simulink model "arm_nonlinear_sim_pi_d_cont_MATLAB_function"  (R2019b)
settings: Solver=ode4  StartTime=0.0  StopTime=3  FixedStep=0.001  RelTol=1e-3
values from neighbouring files (symbols this model uses):
  c = 0.695    [arm_para.m]
  dc = 2    [arm_nonlinear_pi_d_design_MATLAB_function.m]
  g = 9.81    [arm_para.m]
  J = 0.0712    [arm_para.m]
  kD = (d2*gamma_m1^2 - d1*gamma_m1*gamma_m2                    + d0*(gamma_m2^2 - gamma_m1*gamma_m3))/(gamma_m1*gamma_m2)    [arm_nonlinear_pi_d_design_MATLAB_function.m]
  kI = d0/gamma_m1    [arm_nonlinear_pi_d_design_MATLAB_function.m]
  kP = (d2*gamma_m1 - d0*gamma_m3)/(gamma_m1*gamma_m2)    [arm_nonlinear_pi_d_design_MATLAB_function.m]
  l = 0.204    [arm_para.m]
  M = 0.390    (= 0.39)    [arm_para.m]
  rc = rc_deg*(pi/180)    (= 2.09439510239)    [arm_nonlinear_pi_d_design_MATLAB_function.m]
settings Model: Creator=kawata  LastModifiedBy=kawata
settings DataIOCC: ReturnWorkspaceOutputs=off
settings DebuggingCC: ArithmeticOperatorsInVariantConditions=warning
settings SFSimCC: SimUseLocalCustomCode=off  CustomCodeUndefinedFunction=UseInterfaceOnly
settings RTWCC: RTWUseLocalCustomCode=off

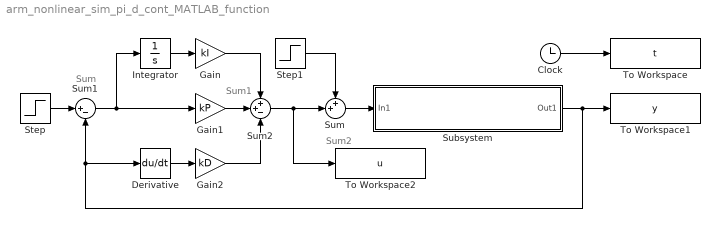
== system arm_nonlinear_sim_pi_d_cont_MATLAB_function ==
  note: Sum1
  note: Sum2
  note: Sum
  Clock : Clock
  Derivative : Derivative
  Gain : Gain  Gain=kI
  Gain1 : Gain  Gain=kP
  Gain2 : Gain  Gain=kD
  Integrator : Integrator
  Step : Step  Time=0  After=rc  SampleTime=0
  Step1 : Step  Time=1.5  After=dc  SampleTime=0
  Subsystem : Subsystem
  Sum : Sum  Inputs=++|
  Sum1 : Sum  Inputs=|+-
  Sum2 : Sum  Inputs=++-
  To Workspace : ToWorkspace  VariableName=t  SampleTime=-1
  To Workspace1 : ToWorkspace  VariableName=y  SampleTime=-1
  To Workspace2 : ToWorkspace  VariableName=u  SampleTime=-1
  wires:
  Subsystem/1(Out1) -> To Workspace1/1, Derivative/1, Sum1/2
  Clock/1 -> To Workspace/1
  Step/1 -> Sum1/1
  Sum/1 -> Subsystem/1(In1)
  Step1/1 -> Sum/1
  Sum2/1 -> To Workspace2/1, Sum/2
  Gain1/1 -> Sum2/2
  Derivative/1 -> Gain2/1
  Gain2/1 -> Sum2/3
  Gain/1 -> Sum2/1
  Sum1/1 -> Gain1/1, Integrator/1
  Integrator/1 -> Gain/1

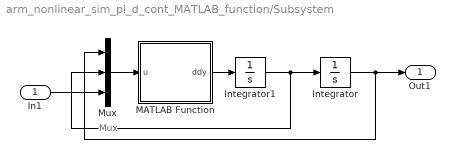
== system arm_nonlinear_sim_pi_d_cont_MATLAB_function/Subsystem ==
  note: Mux
  In1 : Inport
  Integrator : Integrator
  Integrator1 : Integrator
  MATLAB Function : MATLAB Function  TreatAsAtomicUnit=on
  Mux : Mux  Inputs=3
  Out1 : Outport  VectorParamsAs1DForOutWhenUnconnected=off
  wires:
  Mux/1 -> MATLAB Function/1(u)
  MATLAB Function/1(ddy) -> Integrator1/1
  Integrator1/1 -> Mux/2, Integrator/1
  Integrator/1 -> Out1/1, Mux/1
  In1/1 -> Mux/3

== matlab function arm_nonlinear_sim_pi_d_cont_MATLAB_function/Subsystem/MATLAB Function ==
  data: u input; ddy output; M parameter; g parameter; l parameter; c parameter; J parameter
% https://blogs.mathworks.com/japan-community/2021/04/15/matlab-function-block/?from=jp
% にあるように，MATLAB エディタの「データの編集」で M, g, l, c, J の 
% 「Scope」の設定を「Input」から「Parameter」に変更
% （「スコープ」の設定を「入力」から「パラメータ」に変更）

function ddy = fcn(u,M,g,l,c,J)

ddy = (u(3) - M*g*l*sin(u(1)) - c*u(2))/J;
